simulink model "formationControl"  (Simulink 7.0)
settings: Solver=ode45  StartTime=0.0  StopTime=1  RelTol=1e-5
libraries: simulink x1
settings Model: Creator=wizest  LastModifiedBy=wizest

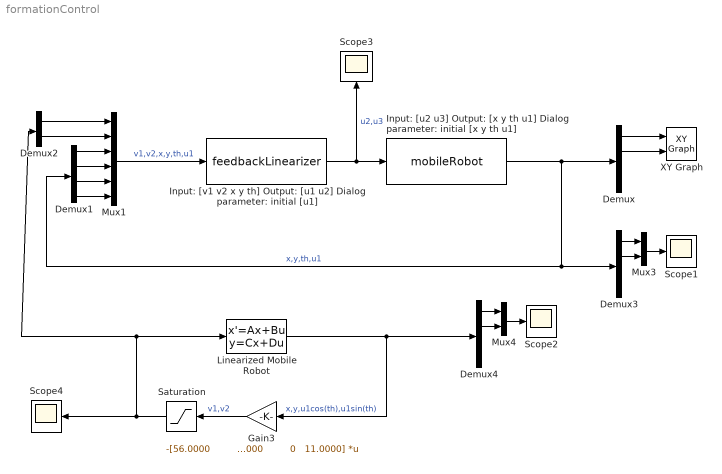
== system formationControl ==
  Demux{,1,3..4} (4 alike) : Demux
  Demux2 : Demux  Outputs=2
  Gain3 : Gain  Orientation=left  Gain="-[56.0000         0   15.0000         0;       0  30.0000         0   11.0000]"  Multiplication=Matrix(K*u) (u vector)  ParameterDataType=sfix(16)  ParameterScaling=2^0  OutDataType=sfix(16)  OutScaling=2^0
  Input: [u2 u3] Output: [x y th u1] Dialog parameter: initial [x y th u1] : M-S-Function  FunctionName=mobileRobot  Parameters=[5 5 1 1]
  Input: [v1 v2 x y th] Output: [u1 u2] Dialog parameter: initial [u1] : M-S-Function  FunctionName=feedbackLinearizer  Parameters=0
  Linearized Mobile Robot : StateSpace  A=[0 0 1 0; 0 0 0 1; 0 0 0 0; 0 0 0 0]  B=[0 0; 0 0; 1 0; 0 1]  C=eye(4)  D=[0 0;0 0 ;0 0;0 0]  X0=[5 5 (1)*cos(1) (1)*sin(1)]
  Mux1 : Mux  Inputs=6
  Mux3 : Mux  Inputs=2
  Mux4 : Mux  Inputs=2
  Saturation : Saturate  Orientation=left  UpperLimit=50  LowerLimit=-50  OutDataType=sfix(16)  OutScaling=2^0
  Scope{1..4} (4 alike) : Scope
      Scope1 settings: TimeRange=1  YMin=0  YMax=6
      Scope2 settings: TimeRange=1  YMin=0  YMax=6  SaveName=ScopeData2
      Scope3 settings: Orientation=up  TimeRange=1  YMin=-100  YMax=400
      Scope4 settings: TimeRange=1  YMin=-60  YMax=40  SaveName=ScopeData3
  XY Graph : simulink/Sinks/XY Graph  SystemSampleTime=-1  xmin=-10  xmax=10  ymin=-10  ymax=10  st=-1
  wires:
  Demux/1 -> XY Graph/1
  Demux/2 -> XY Graph/2
  Mux1/1 -> Input: [v1 v2 x y th] Output: [u1 u2] Dialog parameter: initial [u1]/1  "v1,v2,x,y,th,u1"
  Demux1/1 -> Mux1/3
  Demux1/2 -> Mux1/4
  Input: [v1 v2 x y th] Output: [u1 u2] Dialog parameter: initial [u1]/1 -> Input: [u2 u3] Output: [x y th u1] Dialog parameter: initial [x y th u1]/1, Scope3/1  "u2,u3"
  Input: [u2 u3] Output: [x y th u1] Dialog parameter: initial [x y th u1]/1 -> Demux/1, Demux3/1, Demux1/1  "x,y,th,u1"
  Demux1/3 -> Mux1/5
  Demux1/4 -> Mux1/6
  Linearized Mobile Robot/1 -> Demux4/1, Gain3/1  "x,y,u1cos(th),u1sin(th)"
  Mux4/1 -> Scope2/1
  Demux4/1 -> Mux4/1
  Demux4/2 -> Mux4/2
  Mux3/1 -> Scope1/1
  Demux3/1 -> Mux3/1
  Demux3/2 -> Mux3/2
  Gain3/1 -> Saturation/1  "v1,v2"
  Demux2/1 -> Mux1/1
  Demux2/2 -> Mux1/2
  Saturation/1 -> Linearized Mobile Robot/1, Demux2/1, Scope4/1
